simulink model "nms3D_2021"  (R2021a)
settings: Solver=ode15s  StartTime=0.0  StopTime=2  MaxStep=1e-2  RelTol=1e-2
StartFcn:
  | tic
StopFcn:
  | toc
  | 
  | 
  | %if GimbalLockFlag
  |  % fprintf(2, 'Almost reached Gimbal Lock of IMU. Simulation stopped.\n')
  | %end
  | 
  | %fprintf('Elapsed time: %4.2f sec (%4.2f%% realtime)\n', a, tout(end)/a*100)
values from neighbouring files (symbols this model uses):
  Balance02 = pMod(24:29)    [AssignSimulinkParams.m]    (also in assign_parameters.m = param(26:29))
  Balance13 = pMod(30:35)    [AssignSimulinkParams.m]    (also in assign_parameters.m = param(30:33))
  BalanceTrunk = pMod(22:23)    [AssignSimulinkParams.m]    (also in assign_parameters.m = param(22:23))
  BalanceTrunkLat = param(24:25)    [assign_parameters.m]
  BalanceTrunkLatOld = pMod(43:46)    [AssignSimulinkParams.m]    (also in assign_parameters.m = param(43:46))
  BalanceTrunkOld = param(49:53)    [assign_parameters.m]
  BasisStim = pMod(1:11)    [AssignSimulinkParams.m]    (also in assign_parameters.m = param(1:11))
  CompliantLeg = pMod(12:14)    [AssignSimulinkParams.m]    (also in assign_parameters.m = param(12:14))
  CompliantLegLat = pMod(15)    [AssignSimulinkParams.m]    (also in assign_parameters.m = param(15))
  PreventKneeOverextension = pMod(16:21)    [AssignSimulinkParams.m]    (also in assign_parameters.m = param(16:21))
  SwingCompLatOld = param(47:48)    [assign_parameters.m]
  Target02 = pMod(36:38)    [AssignSimulinkParams.m]    (also in assign_parameters.m = param(34:36))
  Target02_va = pMod(49:54)    [AssignSimulinkParams.m]    (also in assign_parameters.m = param(60:65))
  Target13 = pMod(39:41)    [AssignSimulinkParams.m]    (also in assign_parameters.m = param(37:39))
  Target13_va = pMod(55:60)    [AssignSimulinkParams.m]    (also in assign_parameters.m = param(66:71))
  theta0_world = param(59)    [assign_parameters.m]
  WramameiSL_1000 = readmatrix('WSL_1000_Norm_Sigmoid_MSE_cont.csv')    [nms3D_prep.m]
  ZramameiSL_1000 = readmatrix('ZSL_1000_Norm_Sigmoid_MSE_cont.csv')    [nms3D_prep.m]
undefined symbols (not defined in the file or in its folder): ICs, mParams, X, Y, Z
libraries: nesl_utility x106, sm_lib x87, simulink x70, eeGeneralControl x28, robotmaniplib x14, dspinverses x10, robotcorelib x5, dspmathops x3, vrlib x1, pid_lib x1
(part 8 of 8)

== system nms3D_2021/Supraspinal Level/Subsystem/Stance Leg Control/Stance Leg/Inverse Dynamics Left Leg/Left Leg Ball ==
  note: Here, we select the components we want to control from both the mass matrix and the jacobian. Components from jacobian are used to control the acceleration and components from the mass matrix are used to control the torque
  Config : Inport
  Task : Inport  Port=2
  PD Input : Inport  Port=3
  Enable : EnablePort  ZeroCross=off
  Constant1 : Constant  Value="[0  0]"
  Get Jacobian : robotmaniplib/Get Jacobian  RigidBodyTree=model_left_ball_5dof  EndEffector=EEF  SimulateUsing=Code generation
      settings: SourceProductBaseCode=RO
  Joint Space Mass Matrix : robotmaniplib/Joint Space Mass Matrix  RigidBodyTree=model_left_ball_5dof  SimulateUsing=Code generation
  Matrix Concatenate : Concatenate  Mode=Multidimensional array
  Matrix Multiply1 : Product  Multiplication=Matrix(*)
  Matrix Multiply4 : Product  Multiplication=Matrix(*)
  Mux2 : Mux  Inputs=3
  Pseudoinverse1 : dspinverses/Pseudoinverse  wanterr=off  SimulateUsing=Interpreted execution
      settings: SourceProductBaseCode=DS
  Scope : Scope
  Select entries from jacobian : Selector  NumberOfDimensions=2  InputPortWidth=3  IndexOptions=Index vector (dialog),Index vector (dialog)  Indices=[4 3],[1:6]  OutputSizes=1,1
  Select entries from mass matrix : Selector  NumberOfDimensions=2  InputPortWidth=3  IndexOptions=Index vector (dialog),Index vector (dialog)  Indices=[1 5],[1:6]  OutputSizes=1,1
  Push-Off Left (Ball) : Outport
  wires:
  Matrix Multiply4/1 -> Matrix Multiply1/2
  Config/1 -> Get Jacobian/1, Joint Space Mass Matrix/1
  Select entries from jacobian/1 -> Matrix Concatenate/1
  Pseudoinverse1/1 -> Matrix Multiply4/1
  Matrix Concatenate/1 -> Pseudoinverse1/1
  Select entries from mass matrix/1 -> Matrix Concatenate/2
  Constant1/1 -> Mux2/3
  Mux2/1 -> Matrix Multiply4/2
  Task/1 -> Mux2/1
  Matrix Multiply1/1 -> Push-Off Left (Ball)/1
  Get Jacobian/1 -> Select entries from jacobian/1
  Joint Space Mass Matrix/1 -> Matrix Multiply1/1, Select entries from mass matrix/1
  PD Input/1 -> Scope/1, Mux2/2

== system nms3D_2021/Supraspinal Level/Subsystem/Stance Leg Control/Stance Leg/Subsystem/Right Leg Ball ==
  Config : Inport
  Task : Inport  Port=2
  PD Input : Inport  Port=3
  Enable : EnablePort  ZeroCross=off
  Constant1 : Constant  Value="[0  0]"
  Get Jacobian : robotmaniplib/Get Jacobian  RigidBodyTree=model_right_ball_5dof  EndEffector=EEF  SimulateUsing=Code generation
      settings: SourceProductBaseCode=RO
  Joint Space Mass Matrix : robotmaniplib/Joint Space Mass Matrix  RigidBodyTree=model_right_ball_5dof  SimulateUsing=Code generation
  Matrix Concatenate : Concatenate  Mode=Multidimensional array
  Matrix Multiply1 : Product  Multiplication=Matrix(*)
  Matrix Multiply4 : Product  Multiplication=Matrix(*)
  Mux2 : Mux  Inputs=3
  Pseudoinverse1 : dspinverses/Pseudoinverse  wanterr=off  SimulateUsing=Interpreted execution
      settings: SourceProductBaseCode=DS
  Selector2 : Selector  NumberOfDimensions=2  InputPortWidth=3  IndexOptions=Index vector (dialog),Index vector (dialog)  Indices=[4 3],[1:6]  OutputSizes=1,1
  Selector3 : Selector  NumberOfDimensions=2  InputPortWidth=3  IndexOptions=Index vector (dialog),Index vector (dialog)  Indices=[1 5],[1:6]  OutputSizes=1,1
  Push-Off Right (Ball) : Outport
  wires:
  Matrix Multiply4/1 -> Matrix Multiply1/2
  Config/1 -> Get Jacobian/1, Joint Space Mass Matrix/1
  Selector2/1 -> Matrix Concatenate/1
  Pseudoinverse1/1 -> Matrix Multiply4/1
  Matrix Concatenate/1 -> Pseudoinverse1/1
  Selector3/1 -> Matrix Concatenate/2
  Constant1/1 -> Mux2/3
  Mux2/1 -> Matrix Multiply4/2
  Task/1 -> Mux2/1
  Matrix Multiply1/1 -> Push-Off Right (Ball)/1
  Get Jacobian/1 -> Selector2/1
  Joint Space Mass Matrix/1 -> Matrix Multiply1/1, Selector3/1
  ? -> ?
  PD Input/1 -> Mux2/2

== system nms3D_2021/Supraspinal Level/Subsystem/Swing Leg Control/Compute Acceleration Profiles with Minimal Jerk Approach/ Timer Phase 1/Resettable Subsystem ==
  In1 : Inport
  Enable : EnablePort  ZeroCross=off
  Out1 : Outport
  wires:
  In1/1 -> Out1/1

== system nms3D_2021/Supraspinal Level/Subsystem/Swing Leg Control/Compute Acceleration Profiles with Minimal Jerk Approach/ Timer Phase 2/Resettable Subsystem ==
  In1 : Inport
  Enable : EnablePort  ZeroCross=off
  Out1 : Outport
  wires:
  In1/1 -> Out1/1

== system nms3D_2021/Supraspinal Level/Subsystem/Swing Leg Control/Compute Acceleration Profiles with Minimal Jerk Approach/Minimal jerk Ankle Pitch/Enabled Subsystem ==
  In1 : Inport
  Enable : EnablePort
  Out1 : Outport  VectorParamsAs1DForOutWhenUnconnected=off
  wires:
  In1/1 -> Out1/1

== system nms3D_2021/Supraspinal Level/Subsystem/Swing Leg Control/Compute Acceleration Profiles with Minimal Jerk Approach/Minimal jerk Ankle Pitch/Minimal Jerk ==
  t : Inport
  a [6x1] : Inport  Port=2
  Add : Sum  Inputs=3
  Constant1 : Constant
  Constant3 : Constant  Value=2
  Demux : Demux  Outputs=6
  Divide3 : Product  Inputs=**
  Divide4 : Product  Inputs=**
  Divide5 : Product  Inputs=**
  Gain : Gain  Gain=60
  Gain1 : Gain  Gain=24
  Gain2 : Gain  Gain=6
  Math Function4 : Math  Operator=pow  SaturateOnIntegerOverflow=on
  Terminator : Terminator
  Terminator1 : Terminator
  Terminator2 : Terminator
  j(t) : Outport
  wires:
  a [6x1]/1 -> Demux/1
  Constant3/1 -> Math Function4/2
  Add/1 -> j(t)/1
  Demux/4 -> Divide3/2
  t/1 -> Divide4/1, Math Function4/1
  Demux/5 -> Divide4/2
  Demux/6 -> Divide5/2
  Demux/1 -> Terminator/1
  Demux/2 -> Terminator1/1
  Divide3/1 -> Gain2/1
  Divide4/1 -> Gain1/1
  Divide5/1 -> Gain/1
  Gain/1 -> Add/3
  Gain1/1 -> Add/2
  Gain2/1 -> Add/1
  Math Function4/1 -> Divide5/1
  Constant1/1 -> Divide3/1
  Demux/3 -> Terminator2/1

== system nms3D_2021/Supraspinal Level/Subsystem/Swing Leg Control/Compute Acceleration Profiles with Minimal Jerk Approach/Minimal jerk Ankle Pitch/Minimal Jerk Parameters [Movellan] ==
  x0 : Inport
  dx0 : Inport  Port=2
  ddx0 : Inport  Port=3
  xT : Inport  Port=4
  dxT : Inport  Port=5
  ddxT : Inport  Port=6
  T : Inport  Port=7
  Demux : Demux  Outputs=3
  Gain : Gain  Gain=0.5
  Gain1 : Gain  Gain=3
  Gain2 : Gain  Gain=6
  Gain3 : Gain  Gain=4
  Gain4 : Gain  Gain=12
  Gain5 : Gain  Gain=5
  Gain6 : Gain  Gain=20
  Matrix Multiply : Product  Multiplication=Matrix(*)
  Minus : Sum  Inputs=+---
  Minus1 : Sum  Inputs=+--
  Minus2 : Sum  Inputs=+-
  Mux : Mux  Inputs=6
  Mux{1..4} (4 alike) : Mux  Inputs=3
  Pseudoinverse : dspinverses/Pseudoinverse  wanterr=off  SimulateUsing=Code generation
      settings: SourceProductBaseCode=DS
  T{2..5} (4 alike) : Product  Inputs=**
  b : Concatenate  NumInputs=3  Mode=Multidimensional array  ConcatenateDimension=2
  multiply : Product  Inputs=**
  multiply1 : Product  Inputs=**
  multiply2 : Product  Inputs=**
  a : Outport
  wires:
  xT/1 -> Minus/1
  Minus1/1 -> Mux4/2
  T5/1 -> Mux3/1
  multiply1/1 -> Minus1/3
  Gain5/1 -> Mux3/2
  Demux/2 -> Mux/5
  dxT/1 -> Minus1/1
  Demux/3 -> Mux/6
  b/1 -> Pseudoinverse/1
  multiply2/1 -> Minus/3
  Minus2/1 -> Mux4/3
  Gain/1 -> multiply/1, Mux/3
  multiply/1 -> Minus/4
  ddxT/1 -> Minus2/1
  Gain4/1 -> Mux2/3
  Gain6/1 -> Mux3/3
  x0/1 -> Minus/2, Mux/1
  Mux1/1 -> b/1
  Matrix Multiply/1 -> Demux/1
  ddx0/1 -> Minus2/2, multiply1/1, Gain/1
  T2/1 -> Gain1/1, Gain4/1, T3/1, multiply/2
  Gain2/1 -> Mux1/3
  Mux4/1 -> Matrix Multiply/2
  T4/1 -> Mux2/1, Gain5/1, T5/1
  Minus/1 -> Mux4/1
  Pseudoinverse/1 -> Matrix Multiply/1
  Mux2/1 -> b/2
  Gain3/1 -> Mux2/2
  Mux3/1 -> b/3
  Gain1/1 -> Mux1/2
  T/1 -> multiply2/2, multiply1/2, Gain2/1, T5/2, T4/2, T3/2, T2/2, T2/1
  Demux/1 -> Mux/4
  Mux/1 -> a/1
  T3/1 -> Gain6/1, Gain3/1, Mux1/1, T4/1
  dx0/1 -> multiply2/1, Minus1/2, Mux/2

== system nms3D_2021/Supraspinal Level/Subsystem/Swing Leg Control/Compute Acceleration Profiles with Minimal Jerk Approach/Minimal jerk Ankle Roll/Enabled Subsystem ==
  In1 : Inport
  Enable : EnablePort
  Out1 : Outport  VectorParamsAs1DForOutWhenUnconnected=off
  wires:
  In1/1 -> Out1/1

== system nms3D_2021/Supraspinal Level/Subsystem/Swing Leg Control/Compute Acceleration Profiles with Minimal Jerk Approach/Minimal jerk Ankle Roll/Minimal Jerk ==
  t : Inport
  a [6x1] : Inport  Port=2
  Add : Sum  Inputs=3
  Constant1 : Constant
  Constant3 : Constant  Value=2
  Demux : Demux  Outputs=6
  Divide3 : Product  Inputs=**
  Divide4 : Product  Inputs=**
  Divide5 : Product  Inputs=**
  Gain : Gain  Gain=60
  Gain1 : Gain  Gain=24
  Gain2 : Gain  Gain=6
  Math Function4 : Math  Operator=pow  SaturateOnIntegerOverflow=on
  Terminator : Terminator
  Terminator1 : Terminator
  Terminator2 : Terminator
  j(t) : Outport
  wires:
  a [6x1]/1 -> Demux/1
  Constant3/1 -> Math Function4/2
  Add/1 -> j(t)/1
  Demux/4 -> Divide3/2
  t/1 -> Divide4/1, Math Function4/1
  Demux/5 -> Divide4/2
  Demux/6 -> Divide5/2
  Demux/1 -> Terminator/1
  Demux/2 -> Terminator1/1
  Divide3/1 -> Gain2/1
  Divide4/1 -> Gain1/1
  Divide5/1 -> Gain/1
  Gain/1 -> Add/3
  Gain1/1 -> Add/2
  Gain2/1 -> Add/1
  Math Function4/1 -> Divide5/1
  Constant1/1 -> Divide3/1
  Demux/3 -> Terminator2/1

== system nms3D_2021/Supraspinal Level/Subsystem/Swing Leg Control/Compute Acceleration Profiles with Minimal Jerk Approach/Minimal jerk Ankle Roll/Minimal Jerk Parameters [Movellan] ==
  x0 : Inport
  dx0 : Inport  Port=2
  ddx0 : Inport  Port=3
  xT : Inport  Port=4
  dxT : Inport  Port=5
  ddxT : Inport  Port=6
  T : Inport  Port=7
  Demux : Demux  Outputs=3
  Gain : Gain  Gain=0.5
  Gain1 : Gain  Gain=3
  Gain2 : Gain  Gain=6
  Gain3 : Gain  Gain=4
  Gain4 : Gain  Gain=12
  Gain5 : Gain  Gain=5
  Gain6 : Gain  Gain=20
  Matrix Multiply : Product  Multiplication=Matrix(*)
  Minus : Sum  Inputs=+---
  Minus1 : Sum  Inputs=+--
  Minus2 : Sum  Inputs=+-
  Mux : Mux  Inputs=6
  Mux{1..4} (4 alike) : Mux  Inputs=3
  Pseudoinverse : dspinverses/Pseudoinverse  wanterr=off  SimulateUsing=Code generation
      settings: SourceProductBaseCode=DS
  T{2..5} (4 alike) : Product  Inputs=**
  b : Concatenate  NumInputs=3  Mode=Multidimensional array  ConcatenateDimension=2
  multiply : Product  Inputs=**
  multiply1 : Product  Inputs=**
  multiply2 : Product  Inputs=**
  a : Outport
  wires:
  xT/1 -> Minus/1
  Minus1/1 -> Mux4/2
  T5/1 -> Mux3/1
  multiply1/1 -> Minus1/3
  Gain5/1 -> Mux3/2
  Demux/2 -> Mux/5
  dxT/1 -> Minus1/1
  Demux/3 -> Mux/6
  b/1 -> Pseudoinverse/1
  multiply2/1 -> Minus/3
  Minus2/1 -> Mux4/3
  Gain/1 -> multiply/1, Mux/3
  multiply/1 -> Minus/4
  ddxT/1 -> Minus2/1
  Gain4/1 -> Mux2/3
  Gain6/1 -> Mux3/3
  x0/1 -> Minus/2, Mux/1
  Mux1/1 -> b/1
  Matrix Multiply/1 -> Demux/1
  ddx0/1 -> Minus2/2, multiply1/1, Gain/1
  T2/1 -> Gain1/1, Gain4/1, T3/1, multiply/2
  Gain2/1 -> Mux1/3
  Mux4/1 -> Matrix Multiply/2
  T4/1 -> Mux2/1, Gain5/1, T5/1
  Minus/1 -> Mux4/1
  Pseudoinverse/1 -> Matrix Multiply/1
  Mux2/1 -> b/2
  Gain3/1 -> Mux2/2
  Mux3/1 -> b/3
  Gain1/1 -> Mux1/2
  T/1 -> multiply2/2, multiply1/2, Gain2/1, T5/2, T4/2, T3/2, T2/2, T2/1
  Demux/1 -> Mux/4
  Mux/1 -> a/1
  T3/1 -> Gain6/1, Gain3/1, Mux1/1, T4/1
  dx0/1 -> multiply2/1, Minus1/2, Mux/2

== system nms3D_2021/Supraspinal Level/Subsystem/Swing Leg Control/Compute Acceleration Profiles with Minimal Jerk Approach/Minimal jerk Hip Pitch1/Enabled Subsystem ==
  In1 : Inport
  Enable : EnablePort
  Out1 : Outport  VectorParamsAs1DForOutWhenUnconnected=off
  wires:
  In1/1 -> Out1/1

== system nms3D_2021/Supraspinal Level/Subsystem/Swing Leg Control/Compute Acceleration Profiles with Minimal Jerk Approach/Minimal jerk Hip Pitch1/Minimal Jerk ==
  t : Inport
  a [6x1] : Inport  Port=2
  Add : Sum  Inputs=3
  Constant1 : Constant
  Constant3 : Constant  Value=2
  Demux : Demux  Outputs=6
  Divide3 : Product  Inputs=**
  Divide4 : Product  Inputs=**
  Divide5 : Product  Inputs=**
  Gain : Gain  Gain=60
  Gain1 : Gain  Gain=24
  Gain2 : Gain  Gain=6
  Math Function4 : Math  Operator=pow  SaturateOnIntegerOverflow=on
  Terminator : Terminator
  Terminator1 : Terminator
  Terminator2 : Terminator
  j(t) : Outport
  wires:
  a [6x1]/1 -> Demux/1
  Constant3/1 -> Math Function4/2
  Add/1 -> j(t)/1
  Demux/4 -> Divide3/2
  t/1 -> Divide4/1, Math Function4/1
  Demux/5 -> Divide4/2
  Demux/6 -> Divide5/2
  Demux/1 -> Terminator/1
  Demux/2 -> Terminator1/1
  Divide3/1 -> Gain2/1
  Divide4/1 -> Gain1/1
  Divide5/1 -> Gain/1
  Gain/1 -> Add/3
  Gain1/1 -> Add/2
  Gain2/1 -> Add/1
  Math Function4/1 -> Divide5/1
  Constant1/1 -> Divide3/1
  Demux/3 -> Terminator2/1

== system nms3D_2021/Supraspinal Level/Subsystem/Swing Leg Control/Compute Acceleration Profiles with Minimal Jerk Approach/Minimal jerk Hip Pitch1/Minimal Jerk Parameters [Movellan] ==
  x0 : Inport
  dx0 : Inport  Port=2
  ddx0 : Inport  Port=3
  xT : Inport  Port=4
  dxT : Inport  Port=5
  ddxT : Inport  Port=6
  T : Inport  Port=7
  Demux : Demux  Outputs=3
  Gain : Gain  Gain=0.5
  Gain1 : Gain  Gain=3
  Gain2 : Gain  Gain=6
  Gain3 : Gain  Gain=4
  Gain4 : Gain  Gain=12
  Gain5 : Gain  Gain=5
  Gain6 : Gain  Gain=20
  Matrix Multiply : Product  Multiplication=Matrix(*)
  Minus : Sum  Inputs=+---
  Minus1 : Sum  Inputs=+--
  Minus2 : Sum  Inputs=+-
  Mux : Mux  Inputs=6
  Mux{1..4} (4 alike) : Mux  Inputs=3
  Pseudoinverse : dspinverses/Pseudoinverse  wanterr=off  SimulateUsing=Code generation
      settings: SourceProductBaseCode=DS
  T{2..5} (4 alike) : Product  Inputs=**
  b : Concatenate  NumInputs=3  Mode=Multidimensional array  ConcatenateDimension=2
  multiply : Product  Inputs=**
  multiply1 : Product  Inputs=**
  multiply2 : Product  Inputs=**
  a : Outport
  wires:
  xT/1 -> Minus/1
  Minus1/1 -> Mux4/2
  T5/1 -> Mux3/1
  multiply1/1 -> Minus1/3
  Gain5/1 -> Mux3/2
  Demux/2 -> Mux/5
  dxT/1 -> Minus1/1
  Demux/3 -> Mux/6
  b/1 -> Pseudoinverse/1
  multiply2/1 -> Minus/3
  Minus2/1 -> Mux4/3
  Gain/1 -> multiply/1, Mux/3
  multiply/1 -> Minus/4
  ddxT/1 -> Minus2/1
  Gain4/1 -> Mux2/3
  Gain6/1 -> Mux3/3
  x0/1 -> Minus/2, Mux/1
  Mux1/1 -> b/1
  Matrix Multiply/1 -> Demux/1
  ddx0/1 -> Minus2/2, multiply1/1, Gain/1
  T2/1 -> Gain1/1, Gain4/1, T3/1, multiply/2
  Gain2/1 -> Mux1/3
  Mux4/1 -> Matrix Multiply/2
  T4/1 -> Mux2/1, Gain5/1, T5/1
  Minus/1 -> Mux4/1
  Pseudoinverse/1 -> Matrix Multiply/1
  Mux2/1 -> b/2
  Gain3/1 -> Mux2/2
  Mux3/1 -> b/3
  Gain1/1 -> Mux1/2
  T/1 -> multiply2/2, multiply1/2, Gain2/1, T5/2, T4/2, T3/2, T2/2, T2/1
  Demux/1 -> Mux/4
  Mux/1 -> a/1
  T3/1 -> Gain6/1, Gain3/1, Mux1/1, T4/1
  dx0/1 -> multiply2/1, Minus1/2, Mux/2

== system nms3D_2021/Supraspinal Level/Subsystem/Swing Leg Control/Compute Acceleration Profiles with Minimal Jerk Approach/Minimal jerk Hip Pitch2/Enabled Subsystem ==
  In1 : Inport
  Enable : EnablePort
  Out1 : Outport  VectorParamsAs1DForOutWhenUnconnected=off
  wires:
  In1/1 -> Out1/1

== system nms3D_2021/Supraspinal Level/Subsystem/Swing Leg Control/Compute Acceleration Profiles with Minimal Jerk Approach/Minimal jerk Hip Pitch2/Minimal Jerk ==
  t : Inport
  a [6x1] : Inport  Port=2
  Add : Sum  Inputs=3
  Constant1 : Constant
  Constant3 : Constant  Value=2
  Demux : Demux  Outputs=6
  Divide3 : Product  Inputs=**
  Divide4 : Product  Inputs=**
  Divide5 : Product  Inputs=**
  Gain : Gain  Gain=60
  Gain1 : Gain  Gain=24
  Gain2 : Gain  Gain=6
  Math Function4 : Math  Operator=pow  SaturateOnIntegerOverflow=on
  Terminator : Terminator
  Terminator1 : Terminator
  Terminator2 : Terminator
  j(t) : Outport
  wires:
  a [6x1]/1 -> Demux/1
  Constant3/1 -> Math Function4/2
  Add/1 -> j(t)/1
  Demux/4 -> Divide3/2
  t/1 -> Divide4/1, Math Function4/1
  Demux/5 -> Divide4/2
  Demux/6 -> Divide5/2
  Demux/1 -> Terminator/1
  Demux/2 -> Terminator1/1
  Divide3/1 -> Gain2/1
  Divide4/1 -> Gain1/1
  Divide5/1 -> Gain/1
  Gain/1 -> Add/3
  Gain1/1 -> Add/2
  Gain2/1 -> Add/1
  Math Function4/1 -> Divide5/1
  Constant1/1 -> Divide3/1
  Demux/3 -> Terminator2/1

== system nms3D_2021/Supraspinal Level/Subsystem/Swing Leg Control/Compute Acceleration Profiles with Minimal Jerk Approach/Minimal jerk Hip Pitch2/Minimal Jerk Parameters [Movellan] ==
  x0 : Inport
  dx0 : Inport  Port=2
  ddx0 : Inport  Port=3
  xT : Inport  Port=4
  dxT : Inport  Port=5
  ddxT : Inport  Port=6
  T : Inport  Port=7
  Demux : Demux  Outputs=3
  Gain : Gain  Gain=0.5
  Gain1 : Gain  Gain=3
  Gain2 : Gain  Gain=6
  Gain3 : Gain  Gain=4
  Gain4 : Gain  Gain=12
  Gain5 : Gain  Gain=5
  Gain6 : Gain  Gain=20
  Matrix Multiply : Product  Multiplication=Matrix(*)
  Minus : Sum  Inputs=+---
  Minus1 : Sum  Inputs=+--
  Minus2 : Sum  Inputs=+-
  Mux : Mux  Inputs=6
  Mux{1..4} (4 alike) : Mux  Inputs=3
  Pseudoinverse : dspinverses/Pseudoinverse  wanterr=off  SimulateUsing=Code generation
      settings: SourceProductBaseCode=DS
  T{2..5} (4 alike) : Product  Inputs=**
  b : Concatenate  NumInputs=3  Mode=Multidimensional array  ConcatenateDimension=2
  multiply : Product  Inputs=**
  multiply1 : Product  Inputs=**
  multiply2 : Product  Inputs=**
  a : Outport
  wires:
  xT/1 -> Minus/1
  Minus1/1 -> Mux4/2
  T5/1 -> Mux3/1
  multiply1/1 -> Minus1/3
  Gain5/1 -> Mux3/2
  Demux/2 -> Mux/5
  dxT/1 -> Minus1/1
  Demux/3 -> Mux/6
  b/1 -> Pseudoinverse/1
  multiply2/1 -> Minus/3
  Minus2/1 -> Mux4/3
  Gain/1 -> multiply/1, Mux/3
  multiply/1 -> Minus/4
  ddxT/1 -> Minus2/1
  Gain4/1 -> Mux2/3
  Gain6/1 -> Mux3/3
  x0/1 -> Minus/2, Mux/1
  Mux1/1 -> b/1
  Matrix Multiply/1 -> Demux/1
  ddx0/1 -> Minus2/2, multiply1/1, Gain/1
  T2/1 -> Gain1/1, Gain4/1, T3/1, multiply/2
  Gain2/1 -> Mux1/3
  Mux4/1 -> Matrix Multiply/2
  T4/1 -> Mux2/1, Gain5/1, T5/1
  Minus/1 -> Mux4/1
  Pseudoinverse/1 -> Matrix Multiply/1
  Mux2/1 -> b/2
  Gain3/1 -> Mux2/2
  Mux3/1 -> b/3
  Gain1/1 -> Mux1/2
  T/1 -> multiply2/2, multiply1/2, Gain2/1, T5/2, T4/2, T3/2, T2/2, T2/1
  Demux/1 -> Mux/4
  Mux/1 -> a/1
  T3/1 -> Gain6/1, Gain3/1, Mux1/1, T4/1
  dx0/1 -> multiply2/1, Minus1/2, Mux/2

== system nms3D_2021/Supraspinal Level/Subsystem/Swing Leg Control/Compute Acceleration Profiles with Minimal Jerk Approach/Minimal jerk Hip Pitch3/Enabled Subsystem ==
  In1 : Inport
  Enable : EnablePort
  Out1 : Outport  VectorParamsAs1DForOutWhenUnconnected=off
  wires:
  In1/1 -> Out1/1

== system nms3D_2021/Supraspinal Level/Subsystem/Swing Leg Control/Compute Acceleration Profiles with Minimal Jerk Approach/Minimal jerk Hip Pitch3/Minimal Jerk ==
  t : Inport
  a [6x1] : Inport  Port=2
  Add : Sum  Inputs=3
  Constant1 : Constant
  Constant3 : Constant  Value=2
  Demux : Demux  Outputs=6
  Divide3 : Product  Inputs=**
  Divide4 : Product  Inputs=**
  Divide5 : Product  Inputs=**
  Gain : Gain  Gain=60
  Gain1 : Gain  Gain=24
  Gain2 : Gain  Gain=6
  Math Function4 : Math  Operator=pow  SaturateOnIntegerOverflow=on
  Terminator : Terminator
  Terminator1 : Terminator
  Terminator2 : Terminator
  j(t) : Outport
  wires:
  a [6x1]/1 -> Demux/1
  Constant3/1 -> Math Function4/2
  Add/1 -> j(t)/1
  Demux/4 -> Divide3/2
  t/1 -> Divide4/1, Math Function4/1
  Demux/5 -> Divide4/2
  Demux/6 -> Divide5/2
  Demux/1 -> Terminator/1
  Demux/2 -> Terminator1/1
  Divide3/1 -> Gain2/1
  Divide4/1 -> Gain1/1
  Divide5/1 -> Gain/1
  Gain/1 -> Add/3
  Gain1/1 -> Add/2
  Gain2/1 -> Add/1
  Math Function4/1 -> Divide5/1
  Constant1/1 -> Divide3/1
  Demux/3 -> Terminator2/1

== system nms3D_2021/Supraspinal Level/Subsystem/Swing Leg Control/Compute Acceleration Profiles with Minimal Jerk Approach/Minimal jerk Hip Pitch3/Minimal Jerk Parameters [Movellan] ==
  x0 : Inport
  dx0 : Inport  Port=2
  ddx0 : Inport  Port=3
  xT : Inport  Port=4
  dxT : Inport  Port=5
  ddxT : Inport  Port=6
  T : Inport  Port=7
  Demux : Demux  Outputs=3
  Gain : Gain  Gain=0.5
  Gain1 : Gain  Gain=3
  Gain2 : Gain  Gain=6
  Gain3 : Gain  Gain=4
  Gain4 : Gain  Gain=12
  Gain5 : Gain  Gain=5
  Gain6 : Gain  Gain=20
  Matrix Multiply : Product  Multiplication=Matrix(*)
  Minus : Sum  Inputs=+---
  Minus1 : Sum  Inputs=+--
  Minus2 : Sum  Inputs=+-
  Mux : Mux  Inputs=6
  Mux{1..4} (4 alike) : Mux  Inputs=3
  Pseudoinverse : dspinverses/Pseudoinverse  wanterr=off  SimulateUsing=Code generation
      settings: SourceProductBaseCode=DS
  T{2..5} (4 alike) : Product  Inputs=**
  b : Concatenate  NumInputs=3  Mode=Multidimensional array  ConcatenateDimension=2
  multiply : Product  Inputs=**
  multiply1 : Product  Inputs=**
  multiply2 : Product  Inputs=**
  a : Outport
  wires:
  xT/1 -> Minus/1
  Minus1/1 -> Mux4/2
  T5/1 -> Mux3/1
  multiply1/1 -> Minus1/3
  Gain5/1 -> Mux3/2
  Demux/2 -> Mux/5
  dxT/1 -> Minus1/1
  Demux/3 -> Mux/6
  b/1 -> Pseudoinverse/1
  multiply2/1 -> Minus/3
  Minus2/1 -> Mux4/3
  Gain/1 -> multiply/1, Mux/3
  multiply/1 -> Minus/4
  ddxT/1 -> Minus2/1
  Gain4/1 -> Mux2/3
  Gain6/1 -> Mux3/3
  x0/1 -> Minus/2, Mux/1
  Mux1/1 -> b/1
  Matrix Multiply/1 -> Demux/1
  ddx0/1 -> Minus2/2, multiply1/1, Gain/1
  T2/1 -> Gain1/1, Gain4/1, T3/1, multiply/2
  Gain2/1 -> Mux1/3
  Mux4/1 -> Matrix Multiply/2
  T4/1 -> Mux2/1, Gain5/1, T5/1
  Minus/1 -> Mux4/1
  Pseudoinverse/1 -> Matrix Multiply/1
  Mux2/1 -> b/2
  Gain3/1 -> Mux2/2
  Mux3/1 -> b/3
  Gain1/1 -> Mux1/2
  T/1 -> multiply2/2, multiply1/2, Gain2/1, T5/2, T4/2, T3/2, T2/2, T2/1
  Demux/1 -> Mux/4
  Mux/1 -> a/1
  T3/1 -> Gain6/1, Gain3/1, Mux1/1, T4/1
  dx0/1 -> multiply2/1, Minus1/2, Mux/2

== system nms3D_2021/Supraspinal Level/Subsystem/Swing Leg Control/Compute Acceleration Profiles with Minimal Jerk Approach/Minimal jerk Hip Roll4/Minimal Jerk ==
  t : Inport
  a [6x1] : Inport  Port=2
  Add : Sum  Inputs=3
  Constant1 : Constant
  Constant3 : Constant  Value=2
  Demux : Demux  Outputs=6
  Divide3 : Product  Inputs=**
  Divide4 : Product  Inputs=**
  Divide5 : Product  Inputs=**
  Gain : Gain  Gain=60
  Gain1 : Gain  Gain=24
  Gain2 : Gain  Gain=6
  Math Function4 : Math  Operator=pow  SaturateOnIntegerOverflow=on
  Terminator : Terminator
  Terminator1 : Terminator
  Terminator2 : Terminator
  j(t) : Outport
  wires:
  a [6x1]/1 -> Demux/1
  Constant3/1 -> Math Function4/2
  Add/1 -> j(t)/1
  Demux/4 -> Divide3/2
  t/1 -> Divide4/1, Math Function4/1
  Demux/5 -> Divide4/2
  Demux/6 -> Divide5/2
  Demux/1 -> Terminator/1
  Demux/2 -> Terminator1/1
  Divide3/1 -> Gain2/1
  Divide4/1 -> Gain1/1
  Divide5/1 -> Gain/1
  Gain/1 -> Add/3
  Gain1/1 -> Add/2
  Gain2/1 -> Add/1
  Math Function4/1 -> Divide5/1
  Constant1/1 -> Divide3/1
  Demux/3 -> Terminator2/1

== system nms3D_2021/Supraspinal Level/Subsystem/Swing Leg Control/Compute Acceleration Profiles with Minimal Jerk Approach/Minimal jerk Hip Roll4/Minimal Jerk Parameters[Movellan] ==
  x0 : Inport
  dx0 : Inport  Port=2
  ddx0 : Inport  Port=3
  xT : Inport  Port=4
  dxT : Inport  Port=5
  ddxT : Inport  Port=6
  T : Inport  Port=7
  Demux : Demux  Outputs=3
  Gain : Gain  Gain=0.5
  Gain1 : Gain  Gain=3
  Gain2 : Gain  Gain=6
  Gain3 : Gain  Gain=4
  Gain4 : Gain  Gain=12
  Gain5 : Gain  Gain=5
  Gain6 : Gain  Gain=20
  Matrix Multiply : Product  Multiplication=Matrix(*)
  Minus : Sum  Inputs=+---
  Minus1 : Sum  Inputs=+--
  Minus2 : Sum  Inputs=+-
  Mux : Mux  Inputs=6
  Mux{1..4} (4 alike) : Mux  Inputs=3
  Pseudoinverse : dspinverses/Pseudoinverse  wanterr=off  SimulateUsing=Code generation
      settings: SourceProductBaseCode=DS
  T{2..5} (4 alike) : Product  Inputs=**
  b : Concatenate  NumInputs=3  Mode=Multidimensional array  ConcatenateDimension=2
  multiply : Product  Inputs=**
  multiply1 : Product  Inputs=**
  multiply2 : Product  Inputs=**
  a : Outport
  wires:
  xT/1 -> Minus/1
  Minus1/1 -> Mux4/2
  T5/1 -> Mux3/1
  multiply1/1 -> Minus1/3
  Gain5/1 -> Mux3/2
  Demux/2 -> Mux/5
  dxT/1 -> Minus1/1
  Demux/3 -> Mux/6
  b/1 -> Pseudoinverse/1
  multiply2/1 -> Minus/3
  Minus2/1 -> Mux4/3
  Gain/1 -> multiply/1, Mux/3
  multiply/1 -> Minus/4
  ddxT/1 -> Minus2/1
  Gain4/1 -> Mux2/3
  Gain6/1 -> Mux3/3
  x0/1 -> Minus/2, Mux/1
  Mux1/1 -> b/1
  Matrix Multiply/1 -> Demux/1
  ddx0/1 -> Minus2/2, multiply1/1, Gain/1
  T2/1 -> Gain1/1, Gain4/1, T3/1, multiply/2
  Gain2/1 -> Mux1/3
  Mux4/1 -> Matrix Multiply/2
  T4/1 -> Mux2/1, Gain5/1, T5/1
  Minus/1 -> Mux4/1
  Pseudoinverse/1 -> Matrix Multiply/1
  Mux2/1 -> b/2
  Gain3/1 -> Mux2/2
  Mux3/1 -> b/3
  Gain1/1 -> Mux1/2
  T/1 -> multiply2/2, multiply1/2, Gain2/1, T5/2, T4/2, T3/2, T2/2, T2/1
  Demux/1 -> Mux/4
  Mux/1 -> a/1
  T3/1 -> Gain6/1, Gain3/1, Mux1/1, T4/1
  dx0/1 -> multiply2/1, Minus1/2, Mux/2

== system nms3D_2021/Supraspinal Level/Subsystem/Swing Leg Control/Compute Target States/Balance Control saggital/Enabled Subsystem ==
  CoM Vel : Inport
  Trigger : TriggerPort  TriggerType=falling  VariantControl=Variant  PortDimensions=1
  CoM Vel at Midswing : Outport
  wires:
  CoM Vel/1 -> CoM Vel at Midswing/1

== system nms3D_2021/Supraspinal Level/Subsystem/Swing Leg Control/Inverse Dynamics: Left Leg/Inverse Dynamics/Inverse Dynamics ==
  note: Inverse Dynamics: This block computes the 14 torques (joints(8), body rotation(3) and body translation(3)) needed to generate the desired joint accelerations compensating inertial, velocity depended and gravitational torques at the same time.
  Config : Inport
  JointVel : Inport  Port=2
  Des. JointAccel : Inport  Port=3
  Real JointAccel : Inport  Port=4
  Add : Sum  Inputs=+++
  Constant : Constant  Commented=on  Value=0
  Gravity Torque : robotmaniplib/Gravity Torque  RigidBodyTree=model_swing_left_5dof  SimulateUsing=Code generation
  Joint Space Mass Matrix : robotmaniplib/Joint Space Mass Matrix  RigidBodyTree=model_swing_left_5dof  SimulateUsing=Code generation
  Matrix Multiply : Product  Multiplication=Matrix(*)
  Matrix Multiply1 : Product  Multiplication=Matrix(*)
  Mux3 : Mux  Commented=on  Inputs=2
  Select Body Joint Torques : Selector  InputPortWidth=11  IndexOptions=Index vector (dialog)  Indices=[7:11]  OutputSizes=1
  Select Wrench2 : Selector  InputPortWidth=11  IndexOptions=Index vector (dialog)  Indices=[1 2 3 4 5 6]  OutputSizes=1
  Selector7 : Selector  Commented=on  InputPortWidth=11  IndexOptions=Index vector (dialog)  Indices=[1 2 3 4 5 6 7 8 9 11 10]  OutputSizes=1
  Velocity Product Torque : robotmaniplib/Velocity Product Torque  RigidBodyTree=model_swing_left_5dof  SimulateUsing=Code generation
      settings: SourceProductBaseCode=RO
  Desired Torques : Outport  VectorParamsAs1DForOutWhenUnconnected=off
  Interaction Wrench Left : Outport  Port=2  VectorParamsAs1DForOutWhenUnconnected=off
  wires:
  Add/1 -> Select Body Joint Torques/1
  Select Body Joint Torques/1 -> Desired Torques/1
  Select Wrench2/1 -> Interaction Wrench Left/1
  Joint Space Mass Matrix/1 -> Matrix Multiply1/1, Matrix Multiply/1
  Constant/1 -> Mux3/2
  Config/1 -> Gravity Torque/1, Joint Space Mass Matrix/1, Velocity Product Torque/1
  JointVel/1 -> Velocity Product Torque/2
  Velocity Product Torque/1 -> Add/3
  Gravity Torque/1 -> Add/2
  Matrix Multiply/1 -> Add/1
  Matrix Multiply1/1 -> Select Wrench2/1
  Real JointAccel/1 -> Matrix Multiply1/2
  Mux3/1 -> Selector7/1
  Des. JointAccel/1 -> Matrix Multiply/2, Mux3/1

== system nms3D_2021/Supraspinal Level/Subsystem/Swing Leg Control/Inverse Dynamics: Left Leg/Inverse Dynamics/Inverse Dynamics1 ==
  note: Inverse Dynamics: This block computes the 14 torques (joints(8), body rotation(3) and body translation(3)) needed to generate the desired joint accelerations compensating inertial, velocity depended and gravitational torques at the same time.
  Config : Inport
  JointVel : Inport  Port=2
  Des. JointAccel : Inport  Port=3
  Real JointAccel : Inport  Port=4
  Add : Sum  Inputs=+++
  Constant : Constant  Value=0
  Gravity Torque : robotmaniplib/Gravity Torque  RigidBodyTree=model_swing_left_5dof  SimulateUsing=Code generation
  Joint Space Mass Matrix : robotmaniplib/Joint Space Mass Matrix  RigidBodyTree=model_swing_left_5dof  SimulateUsing=Code generation
  Matrix Multiply : Product  Multiplication=Matrix(*)
  Matrix Multiply1 : Product  Multiplication=Matrix(*)
  Mux{,1..3} (4 alike) : Mux  Inputs=2
  Scope1 : Scope  NumInputPorts=2
  Scope2 : Scope
  Scope3 : Scope
  Scope4 : Scope  NumInputPorts=2
  Scope5 : Scope  NumInputPorts=2
  Select Body Joint Torques : Selector  InputPortWidth=10  IndexOptions=Index vector (dialog)  Indices=[7:10]  OutputSizes=1
  Select Wrench2 : Selector  InputPortWidth=10  IndexOptions=Index vector (dialog)  Indices=[1 2 3 4 5 6]  OutputSizes=1
  Selector{,1,6..7} (4 alike) : Selector  InputPortWidth=11  IndexOptions=Index vector (dialog)  Indices=[1 2 3 4 5 6 7 8 9 11 10]  OutputSizes=1
  Selector{2..5,8..10} (7 alike) : Selector  InputPortWidth=11  IndexOptions=Index vector (dialog)  Indices=[1 2 3 4 5 6 7 8 9 11 ]  OutputSizes=1
  Selector{11..16} (6 alike) : Selector  InputPortWidth=11  IndexOptions=Index vector (dialog)  Indices=[ 7 8 9 10 11 ]  OutputSizes=1
  Velocity Product Torque : robotmaniplib/Velocity Product Torque  RigidBodyTree=model_swing_left_5dof  SimulateUsing=Code generation
      settings: SourceProductBaseCode=RO
  Desired Torques : Outport  VectorParamsAs1DForOutWhenUnconnected=off
  Interaction Wrench Left : Outport  Port=2  VectorParamsAs1DForOutWhenUnconnected=off
  wires:
  Add/1 -> Select Body Joint Torques/1
  Select Body Joint Torques/1 -> Desired Torques/1
  Gravity Torque/1 -> Selector3/1
  Select Wrench2/1 -> Interaction Wrench Left/1
  Matrix Multiply1/1 -> Selector5/1
  Joint Space Mass Matrix/1 -> Matrix Multiply1/1, Matrix Multiply/1
  Matrix Multiply/1 -> Selector4/1
  Velocity Product Torque/1 -> Selector2/1
  Constant/1 -> Mux2/2, Mux3/2, Mux/2, Mux1/2
  Mux/1 -> Selector/1
  Mux1/1 -> Selector1/1
  Config/1 -> Velocity Product Torque/1, Gravity Torque/1, Joint Space Mass Matrix/1, Selector11/1, Selector8/1
  JointVel/1 -> Velocity Product Torque/2, Selector13/1, Selector9/1
  Selector2/1 -> Add/3
  Selector3/1 -> Add/2
  Selector4/1 -> Add/1
  Selector5/1 -> Select Wrench2/1
  Real JointAccel/1 -> Matrix Multiply1/2, Selector15/1, Selector10/1
  Selector7/1 -> Matrix Multiply/2
  Mux3/1 -> Scope2/1, Selector7/1
  Des. JointAccel/1 -> Mux3/1
  Mux2/1 -> Selector6/1
  Selector8/1 -> Mux1/1
  Selector1/1 -> Selector12/1
  Selector/1 -> Selector14/1
  Selector9/1 -> Mux/1
  Selector10/1 -> Mux2/1
  Selector6/1 -> Selector16/1
  Selector11/1 -> Scope4/1
  Selector12/1 -> Scope4/2
  Selector13/1 -> Scope5/2
  Selector14/1 -> Scope5/1
  Selector15/1 -> Scope1/2
  Selector16/1 -> Scope1/1

== system nms3D_2021/Supraspinal Level/Subsystem/Swing Leg Control/Inverse Dynamics: Right Leg/Inverse Dynamics1/Inverse Dynamics ==
  note: Inverse Dynamics: This block computes the 14 torques (joints(8), body rotation(3) and body translation(3)) needed to generate the desired joint accelerations compensating inertial, velocity depended and gravitational torques at the same time.
  Config : Inport
  JointVel : Inport  Port=2
  Des. JointAccel : Inport  Port=3
  Real JointAccel : Inport  Port=4
  Add : Sum  Inputs=+++
  Constant : Constant  Commented=on  Value=0
  Gravity Torque : robotmaniplib/Gravity Torque  RigidBodyTree=model_swing_right_5dof  SimulateUsing=Code generation
  Joint Space Mass Matrix : robotmaniplib/Joint Space Mass Matrix  RigidBodyTree=model_swing_right_5dof  SimulateUsing=Code generation
  Matrix Multiply : Product  Multiplication=Matrix(*)
  Matrix Multiply1 : Product  Multiplication=Matrix(*)
  Mux4 : Mux  Commented=on  Inputs=2
  Select Body Joint Torques : Selector  InputPortWidth=11  IndexOptions=Index vector (dialog)  Indices=[7:11]  OutputSizes=1
  Select Wrench2 : Selector  InputPortWidth=11  IndexOptions=Index vector (dialog)  Indices=[1 2 3 4 5 6]  OutputSizes=1
  Selector3 : Selector  Commented=on  InputPortWidth=11  IndexOptions=Index vector (dialog)  Indices=[1 2 3 4 5 6 7 8 9 11 10]  OutputSizes=1
  Velocity Product Torque : robotmaniplib/Velocity Product Torque  RigidBodyTree=model_swing_right_5dof  SimulateUsing=Code generation
      settings: SourceProductBaseCode=RO
  Desired Torques : Outport  VectorParamsAs1DForOutWhenUnconnected=off
  Interaction Wrench Left : Outport  Port=2  VectorParamsAs1DForOutWhenUnconnected=off
  wires:
  Add/1 -> Select Body Joint Torques/1
  Select Body Joint Torques/1 -> Desired Torques/1
  Select Wrench2/1 -> Interaction Wrench Left/1
  Joint Space Mass Matrix/1 -> Matrix Multiply1/1, Matrix Multiply/1
  Config/1 -> Joint Space Mass Matrix/1, Gravity Torque/1, Velocity Product Torque/1
  JointVel/1 -> Velocity Product Torque/2
  Mux4/1 -> Selector3/1
  Des. JointAccel/1 -> Matrix Multiply/2, Mux4/1
  Real JointAccel/1 -> Matrix Multiply1/2
  Constant/1 -> Mux4/2
  Velocity Product Torque/1 -> Add/3
  Gravity Torque/1 -> Add/2
  Matrix Multiply/1 -> Add/1
  Matrix Multiply1/1 -> Select Wrench2/1

== stateflow chart nms3D_2021/Supraspinal Level/Finite State Machine/Chart ==
  settings: executeAtInitialization=1
  state State0
    entry:
    state0=1;
    state1=0;
    state2=0;
    state3=0;
  state State1
    entry:
    state0=0;
    state1=1;
    state2=0;
    state3=0;
  state State3
    entry:
    state0=0;
    state1=0;
    state2=0;
    state3=1;
  state State2
    entry:
    state0=0;
    state1=0;
    state2=1;
    state3=0;
  (default) -> State0
  State0 -> State1 : after(dt,sec)
  State3 -> State0 : [contact_left]
  State1 -> State2 : [contact_right]
  State2 -> State3 : after(dt,sec)
  data: state0 output; state1 output; state2 output; state3 output; dt input; contact_left input; contact_right input
